simulink model "Even_Odd"  (R2021a)
settings: Solver=FixedStepDiscrete  StartTime=0.0  StopTime=10.0  RelTol=1e-3  EnableMultiTasking=on
settings Model: Creator=top one  LastModifiedBy=top one
settings DataIOCC: ReturnWorkspaceOutputs=off
settings OptimizationCC: DefaultParameterBehavior=Inlined  InlineInvariantSignals=on  EnableMemcpy=off  LifeSpan=1  EfficientTunableParamExpr=on
settings DebuggingCC: UnderspecifiedInitializationDetection=Classic  MergeDetectMultiDrivingBlocksExec=none  SFMachineParentedDataDiag=warning  ArithmeticOperatorsInVariantConditions=warning
settings ModelReferenceCC: PropagateSignalLabelsOutOfModel=off
settings SFSimCC: MATLABDynamicMemAlloc=off  CustomCodeUndefinedFunction=UseInterfaceOnly
settings RTWCC: SystemTargetFile=ert.tlc  GenCodeOnly=on  TemplateMakefile=ert_default_tmf  GenerateReport=on  IncludeHyperlinkInReport=on  LaunchReport=on  GenerateTraceInfo=on  GenerateTraceReport=on  GenerateTraceReportSl=on  GenerateTraceReportSf=on  GenerateTraceReportEml=on
settings CodeAppCC: ForceParamTrailComments=on  IgnoreCustomStorageClasses=off  OperatorAnnotations=on  SimulinkDataObjDesc=on  SFDataObjDesc=on  MATLABFcnDesc=on  InsertBlockDesc=on  StateflowObjectComments=on  MATLABSourceComments=on
settings ERTTargetCC: MultiwordLength=2048  GenerateSampleERTMain=on  InlinedParameterPlacement=NonHierarchical  ERTCustomFileTemplate=example_file_process.tlc

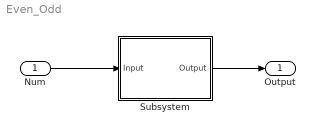
== system Even_Odd ==
  Num : Inport
  Subsystem : Subsystem
  Output : Outport
  wires:
  Num/1 -> Subsystem/1(Input)
  Subsystem/1(Output) -> Output/1

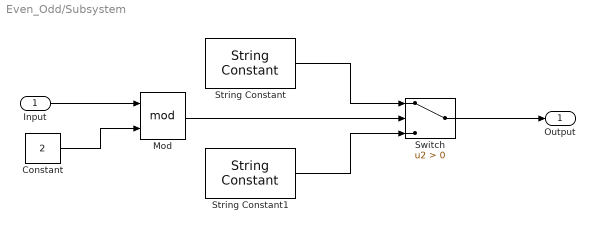
== system Even_Odd/Subsystem ==
  Input : Inport
  Constant : Constant  Value=2
  Mod : Math  Operator=mod  SaturateOnIntegerOverflow=on
  String Constant : StringConstant  String="\"Odd\""
  String Constant1 : StringConstant  String="\"Even\""
  Switch : Switch  Criteria=u2 > Threshold
  Output : Outport
  wires:
  String Constant1/1 -> Switch/3
  Switch/1 -> Output/1
  Input/1 -> Mod/1
  Constant/1 -> Mod/2
  String Constant/1 -> Switch/1
  Mod/1 -> Switch/2
